simulink model "HDL_source"  (R2019a)
settings: Solver=FixedStepDiscrete  StartTime=0.0  StopTime=0.1  RelTol=1e-3
PreLoadFcn:
  | load('visionhdlLaneDetectionInit.mat');
  | 
  | %Birds-Eye View Parameters:
  | T_unreal = [-0.346719845290643,-3.45626583672944e-16,-2.42608110520569e-19;-1.76272742794994,-2.62399506819665,-0.00185184300876343;1283.14845282490,1569.57420684550,1];
  | shiftleft = single([-5,-5,-5,-5,-5,-5,-5,-5,-5,-5,   -5,-4,-2,-2,-2,-2,0,0,0,1,    1,2,3,4,5,6,7,10,11,13,     15,17,20,22,26,30,33,38,42,46]);
  | shiftright = single([-20,-20,-20,-20,-20,-20,-20,-20,-20,-20,    -20,-20,-20,-21,-22,-23,-24,-24,-24,-25,    -26,-27,-28,-29,-30,-32,-33,-35,-37,-39,    -41,-45,-46,-50,-53,-57,-61,-67,-72,-78]);
StartFcn:
  | warning('off','Coder:MATLAB:polyfit_RepeatedPointsOrRescale');
  | warning('off','Coder:MATLAB:rankDeficientMatrix');
StopFcn:
  | warning('on','Coder:MATLAB:polyfit_RepeatedPointsOrRescale');
  | warning('on','Coder:MATLAB:rankDeficientMatrix');
undefined symbols (not defined in the file): gray, h1, imresize, Rec, SDTV
libraries: simulink x31, hdlsllib x19, visionhdlutilities x6, visionhdlstatistics x4, visiongeotforms x3, visionhdlio x2, visiontextngfix x2, visionhdlconversions x1, visionhdlgeotforms x1, visionhdlfilter x1, dspvision x1, visionsinks x1
(part 2 of 3)

== system HDL_source/FPGALaneDetection/Lane Detection Algorithm/ComputeEgoLanes1/FirstPassEgoLane/rightminop6 ==
  val1 : Inport
  val2 : Inport  Port=2
  ind1 : Inport  Port=3
  ind2 : Inport  Port=4
  Delay{,1..5} (6 alike) : Delay  DelayLength=1
  Multiport Switch : MultiPortSwitch  DataPortOrder=Zero-based contiguous  Inputs=2  zeroidx=on
  Multiport Switch1 : MultiPortSwitch  DataPortOrder=Zero-based contiguous  Inputs=2  zeroidx=on
  Relational Operator : RelationalOperator  Operator=<=  OutDataTypeStr=boolean  RndMeth=Simplest
  valmin : Outport
  indmin : Outport  Port=2
  wires:
  val1/1 -> Delay2/1
  Multiport Switch1/1 -> Delay1/1
  val2/1 -> Delay3/1
  ind1/1 -> Delay4/1
  Multiport Switch/1 -> Delay/1
  Relational Operator/1 -> Multiport Switch/1, Multiport Switch1/1
  ind2/1 -> Delay5/1
  Delay/1 -> valmin/1
  Delay1/1 -> indmin/1
  Delay2/1 -> Relational Operator/1, Multiport Switch/3
  Delay3/1 -> Relational Operator/2, Multiport Switch/2
  Delay4/1 -> Multiport Switch1/3
  Delay5/1 -> Multiport Switch1/2

== system HDL_source/FPGALaneDetection/Lane Detection Algorithm/ComputeEgoLanes1/FirstPassEgoLane/rightminop7 ==
  val1 : Inport
  val2 : Inport  Port=2
  ind1 : Inport  Port=3
  ind2 : Inport  Port=4
  Delay{,1..5} (6 alike) : Delay  DelayLength=1
  Multiport Switch : MultiPortSwitch  DataPortOrder=Zero-based contiguous  Inputs=2  zeroidx=on
  Multiport Switch1 : MultiPortSwitch  DataPortOrder=Zero-based contiguous  Inputs=2  zeroidx=on
  Relational Operator : RelationalOperator  Operator=<=  OutDataTypeStr=boolean  RndMeth=Simplest
  valmin : Outport
  indmin : Outport  Port=2
  wires:
  Delay5/1 -> Multiport Switch1/2
  Delay4/1 -> Multiport Switch1/3
  Delay3/1 -> Multiport Switch/2, Relational Operator/2
  Delay2/1 -> Multiport Switch/3, Relational Operator/1
  Delay1/1 -> indmin/1
  Delay/1 -> valmin/1
  ind2/1 -> Delay5/1
  Relational Operator/1 -> Multiport Switch1/1, Multiport Switch/1
  Multiport Switch/1 -> Delay/1
  ind1/1 -> Delay4/1
  val2/1 -> Delay3/1
  Multiport Switch1/1 -> Delay1/1
  val1/1 -> Delay2/1

== system HDL_source/FPGALaneDetection/Lane Detection Algorithm/ComputeEgoLanes1/FirstPassEgoLane/rightminop8 ==
  val1 : Inport
  val2 : Inport  Port=2
  ind1 : Inport  Port=3
  ind2 : Inport  Port=4
  Delay{,1..5} (6 alike) : Delay  DelayLength=1
  Multiport Switch : MultiPortSwitch  DataPortOrder=Zero-based contiguous  Inputs=2  zeroidx=on
  Multiport Switch1 : MultiPortSwitch  DataPortOrder=Zero-based contiguous  Inputs=2  zeroidx=on
  Relational Operator : RelationalOperator  Operator=<=  OutDataTypeStr=boolean  RndMeth=Simplest
  valmin : Outport
  indmin : Outport  Port=2
  wires:
  val1/1 -> Delay2/1
  Multiport Switch1/1 -> Delay1/1
  val2/1 -> Delay3/1
  ind1/1 -> Delay4/1
  Multiport Switch/1 -> Delay/1
  Relational Operator/1 -> Multiport Switch/1, Multiport Switch1/1
  ind2/1 -> Delay5/1
  Delay/1 -> valmin/1
  Delay1/1 -> indmin/1
  Delay2/1 -> Relational Operator/1, Multiport Switch/3
  Delay3/1 -> Relational Operator/2, Multiport Switch/2
  Delay4/1 -> Multiport Switch1/3
  Delay5/1 -> Multiport Switch1/2

== system HDL_source/FPGALaneDetection/Lane Detection Algorithm/ComputeEgoLanes1/FirstPassEgoLane/rightminop9 ==
  val1 : Inport
  val2 : Inport  Port=2
  ind1 : Inport  Port=3
  ind2 : Inport  Port=4
  Delay{,1..5} (6 alike) : Delay  DelayLength=1
  Multiport Switch : MultiPortSwitch  DataPortOrder=Zero-based contiguous  Inputs=2  zeroidx=on
  Multiport Switch1 : MultiPortSwitch  DataPortOrder=Zero-based contiguous  Inputs=2  zeroidx=on
  Relational Operator : RelationalOperator  Operator=<=  OutDataTypeStr=boolean  RndMeth=Simplest
  valmin : Outport
  indmin : Outport  Port=2
  wires:
  Delay5/1 -> Multiport Switch1/2
  Delay4/1 -> Multiport Switch1/3
  Delay3/1 -> Multiport Switch/2, Relational Operator/2
  Delay2/1 -> Multiport Switch/3, Relational Operator/1
  Delay1/1 -> indmin/1
  Delay/1 -> valmin/1
  ind2/1 -> Delay5/1
  Relational Operator/1 -> Multiport Switch1/1, Multiport Switch/1
  Multiport Switch/1 -> Delay/1
  ind1/1 -> Delay4/1
  val2/1 -> Delay3/1
  Multiport Switch1/1 -> Delay1/1
  val1/1 -> Delay2/1

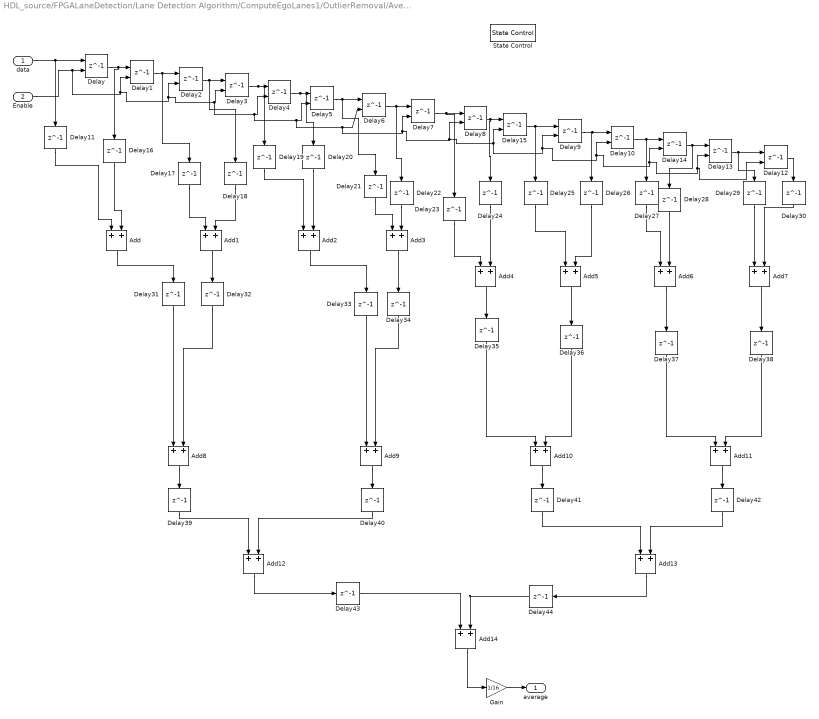
== system HDL_source/FPGALaneDetection/Lane Detection Algorithm/ComputeEgoLanes1/OutlierRemoval/AverageLeftWidth ==
  data : Inport
  Enable : Inport  Port=2
  Add{,1..14} (15 alike) : Sum  OutDataTypeStr=fixdt(1,16,0)
  Delay{,1..10,12..15} (15 alike) : Delay  DelayLength=1  ShowEnablePort=on
      settings: InputPortMap=u0,e6
  Delay{11,16..44} (30 alike) : Delay  DelayLength=1
  Gain : Gain  Gain=1/16
  State Control : StateControl  StateControl=Synchronous
  average : Outport
  wires:
  Delay44/1 -> Add14/2
  Delay43/1 -> Add14/1
  Delay42/1 -> Add13/2
  Delay41/1 -> Add13/1
  Delay40/1 -> Add12/2
  Delay39/1 -> Add12/1
  Delay38/1 -> Add11/2
  Delay37/1 -> Add11/1
  Delay36/1 -> Add10/2
  Delay35/1 -> Add10/1
  Delay34/1 -> Add9/2
  Delay33/1 -> Add9/1
  Delay32/1 -> Add8/2
  Delay31/1 -> Add8/1
  Delay30/1 -> Add7/2
  Delay29/1 -> Add7/1
  Delay28/1 -> Add6/2
  Delay10/1 -> Delay14/1, Delay27/1
  Delay27/1 -> Add6/1
  Delay26/1 -> Add5/2
  Delay25/1 -> Add5/1
  Delay24/1 -> Add4/2
  Delay23/1 -> Add4/1
  Delay22/1 -> Add3/2
  Delay21/1 -> Add3/1
  Delay20/1 -> Add2/2
  Delay19/1 -> Add2/1
  Delay18/1 -> Add1/2
  Delay17/1 -> Add1/1
  Delay16/1 -> Add/2
  Delay11/1 -> Add/1
  Add13/1 -> Delay44/1
  Add12/1 -> Delay43/1
  Add11/1 -> Delay42/1
  Add10/1 -> Delay41/1
  Add9/1 -> Delay40/1
  Add8/1 -> Delay39/1
  Add7/1 -> Delay38/1
  Add6/1 -> Delay37/1
  Add5/1 -> Delay36/1
  Add4/1 -> Delay35/1
  Add3/1 -> Delay34/1
  Add2/1 -> Delay33/1
  Add1/1 -> Delay32/1
  Add/1 -> Delay31/1
  Add14/1 -> Gain/1
  Gain/1 -> average/1
  Delay13/1 -> Delay12/1, Delay29/1
  Delay/1 -> Delay1/1, Delay16/1
  Delay12/1 -> Delay30/1
  Delay14/1 -> Delay13/1, Delay28/1
  Delay9/1 -> Delay10/1, Delay26/1
  Delay15/1 -> Delay9/1, Delay25/1
  Delay8/1 -> Delay15/1, Delay24/1
  Delay7/1 -> Delay8/1, Delay23/1
  Delay6/1 -> Delay7/1, Delay22/1
  Delay5/1 -> Delay6/1, Delay21/1
  Delay4/1 -> Delay20/1, Delay5/1
  Delay3/1 -> Delay4/1, Delay19/1
  Delay2/1 -> Delay3/1, Delay18/1
  Delay1/1 -> Delay2/1, Delay17/1
  Enable/1 -> Delay/2, Delay1/2, Delay2/2, Delay3/2, Delay4/2, Delay5/2, Delay6/2, Delay7/2, Delay8/2, Delay9/2, Delay10/2, Delay14/2, Delay13/2, Delay12/2, Delay15/2
  data/1 -> Delay/1, Delay11/1

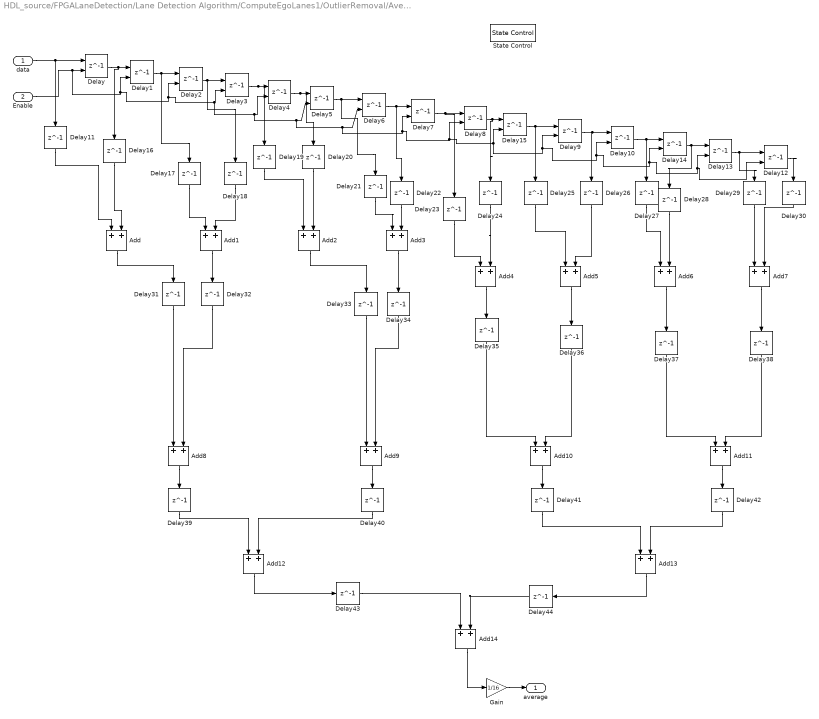
== system HDL_source/FPGALaneDetection/Lane Detection Algorithm/ComputeEgoLanes1/OutlierRemoval/AverageRightWidth ==
  data : Inport
  Enable : Inport  Port=2
  Add{,1..14} (15 alike) : Sum  OutDataTypeStr=fixdt(1,16,0)
  Delay{,1..10,12..15} (15 alike) : Delay  DelayLength=1  ShowEnablePort=on
      settings: InputPortMap=u0,e6
  Delay{11,16..44} (30 alike) : Delay  DelayLength=1
  Gain : Gain  Gain=1/16
  State Control : StateControl  StateControl=Synchronous
  average : Outport
  wires:
  data/1 -> Delay11/1, Delay/1
  Enable/1 -> Delay15/2, Delay12/2, Delay13/2, Delay14/2, Delay10/2, Delay9/2, Delay8/2, Delay7/2, Delay6/2, Delay5/2, Delay4/2, Delay3/2, Delay2/2, Delay1/2, Delay/2
  Delay1/1 -> Delay17/1, Delay2/1
  Delay2/1 -> Delay18/1, Delay3/1
  Delay3/1 -> Delay19/1, Delay4/1
  Delay4/1 -> Delay20/1, Delay5/1
  Delay5/1 -> Delay21/1, Delay6/1
  Delay6/1 -> Delay22/1, Delay7/1
  Delay7/1 -> Delay23/1, Delay8/1
  Delay8/1 -> Delay24/1, Delay15/1
  Delay15/1 -> Delay25/1, Delay9/1
  Delay9/1 -> Delay26/1, Delay10/1
  Delay14/1 -> Delay28/1, Delay13/1
  Delay12/1 -> Delay30/1
  Delay/1 -> Delay16/1, Delay1/1
  Delay13/1 -> Delay29/1, Delay12/1
  Gain/1 -> average/1
  Add14/1 -> Gain/1
  Add/1 -> Delay31/1
  Add1/1 -> Delay32/1
  Add2/1 -> Delay33/1
  Add3/1 -> Delay34/1
  Add4/1 -> Delay35/1
  Add5/1 -> Delay36/1
  Add6/1 -> Delay37/1
  Add7/1 -> Delay38/1
  Add8/1 -> Delay39/1
  Add9/1 -> Delay40/1
  Add10/1 -> Delay41/1
  Add11/1 -> Delay42/1
  Add12/1 -> Delay43/1
  Add13/1 -> Delay44/1
  Delay11/1 -> Add/1
  Delay16/1 -> Add/2
  Delay17/1 -> Add1/1
  Delay18/1 -> Add1/2
  Delay19/1 -> Add2/1
  Delay20/1 -> Add2/2
  Delay21/1 -> Add3/1
  Delay22/1 -> Add3/2
  Delay23/1 -> Add4/1
  Delay24/1 -> Add4/2
  Delay25/1 -> Add5/1
  Delay26/1 -> Add5/2
  Delay27/1 -> Add6/1
  Delay10/1 -> Delay27/1, Delay14/1
  Delay28/1 -> Add6/2
  Delay29/1 -> Add7/1
  Delay30/1 -> Add7/2
  Delay31/1 -> Add8/1
  Delay32/1 -> Add8/2
  Delay33/1 -> Add9/1
  Delay34/1 -> Add9/2
  Delay35/1 -> Add10/1
  Delay36/1 -> Add10/2
  Delay37/1 -> Add11/1
  Delay38/1 -> Add11/2
  Delay39/1 -> Add12/1
  Delay40/1 -> Add12/2
  Delay41/1 -> Add13/1
  Delay42/1 -> Add13/2
  Delay43/1 -> Add14/1
  Delay44/1 -> Add14/2

== system HDL_source/FPGALaneDetection/Lane Detection Algorithm/ComputeEgoLanes1/OutlierRemoval/RemoveOutlier ==
  laneVal : Inport
  offsetVal : Inport  Port=2
  width : Inport  Port=3
  Constant2 : Constant  Value=0  OutDataTypeStr=uint16  SampleTime=-1
  Delay{13..15,17} (4 alike) : Delay  DelayLength=1
  Multiport Switch : MultiPortSwitch  DataPortOrder=Zero-based contiguous  Inputs=2  zeroidx=on
  Relational Operator : RelationalOperator  Operator=<=  OutDataTypeStr=boolean  RndMeth=Simplest
  Inlier : Outport
  wires:
  Delay14/1 -> Multiport Switch/2
  Multiport Switch/1 -> Delay17/1
  Delay15/1 -> Multiport Switch/3
  Relational Operator/1 -> Delay13/1
  offsetVal/1 -> Relational Operator/1
  laneVal/1 -> Delay15/1
  Constant2/1 -> Delay14/1
  Delay13/1 -> Multiport Switch/1
  width/1 -> Relational Operator/2
  Delay17/1 -> Inlier/1

== system HDL_source/FPGALaneDetection/Lane Detection Algorithm/ComputeEgoLanes1/OutlierRemoval/RemoveOutlier1 ==
  laneVal : Inport
  offsetVal : Inport  Port=2
  width : Inport  Port=3
  Constant2 : Constant  Value=0  OutDataTypeStr=uint16  SampleTime=-1
  Delay{13..15,17} (4 alike) : Delay  DelayLength=1
  Multiport Switch : MultiPortSwitch  DataPortOrder=Zero-based contiguous  Inputs=2  zeroidx=on
  Relational Operator : RelationalOperator  Operator=<=  OutDataTypeStr=boolean  RndMeth=Simplest
  Inlier : Outport
  wires:
  Delay17/1 -> Inlier/1
  width/1 -> Relational Operator/2
  Delay13/1 -> Multiport Switch/1
  Constant2/1 -> Delay14/1
  laneVal/1 -> Delay15/1
  offsetVal/1 -> Relational Operator/1
  Relational Operator/1 -> Delay13/1
  Delay15/1 -> Multiport Switch/3
  Multiport Switch/1 -> Delay17/1
  Delay14/1 -> Multiport Switch/2

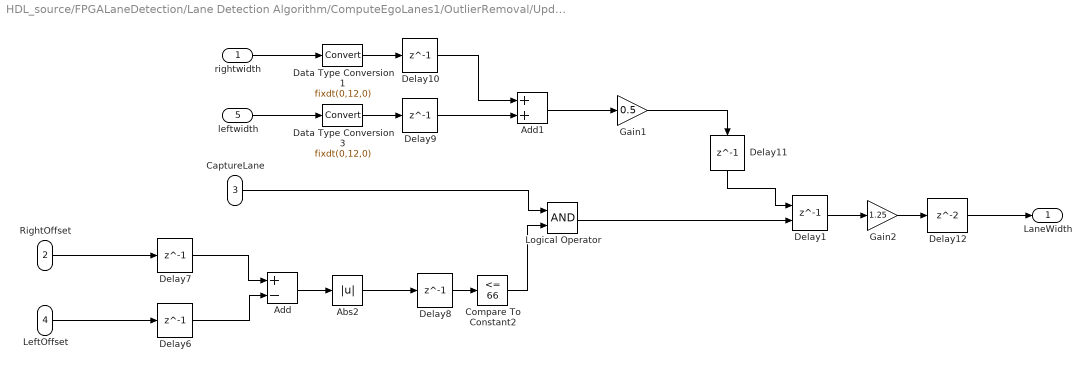
== system HDL_source/FPGALaneDetection/Lane Detection Algorithm/ComputeEgoLanes1/OutlierRemoval/UpdateLaneWidth ==
  rightwidth : Inport
  RightOffset : Inport  Port=2
  CaptureLane : Inport  Port=3
  LeftOffset : Inport  Port=4
  leftwidth : Inport  Port=5
  Abs2 : Abs  OutDataTypeStr=fixdt(0,14,0)
  Add : Sum  Inputs=+-  SaturateOnIntegerOverflow=on
  Add1 : Sum
  Compare To Constant2 : simulink/Logic and Bit Operations/Compare To Constant  relop=<=  const=66  OutDataTypeStr=boolean
  Data Type Conversion1 : DataTypeConversion  OutDataTypeStr=fixdt(0,12,0)  RndMeth=Round  SaturateOnIntegerOverflow=on
  Data Type Conversion3 : DataTypeConversion  OutDataTypeStr=fixdt(0,12,0)  RndMeth=Round  SaturateOnIntegerOverflow=on
  Delay1 : Delay  DelayLength=1  ShowEnablePort=on
      settings: InputPortMap=u0,e6
  Delay{6..11} (6 alike) : Delay  DelayLength=1
  Delay12 : Delay
  Gain1 : Gain  Gain=0.5  OutDataTypeStr=fixdt(0,16,0)  RndMeth=Round  SaturateOnIntegerOverflow=on
  Gain2 : Gain  Gain=1.25  OutDataTypeStr=fixdt(1,18,0)
  Logical Operator : Logic  AllPortsSameDT=off  OutDataTypeStr=boolean
  LaneWidth : Outport
  wires:
  Compare To Constant2/1 -> Logical Operator/2
  Gain1/1 -> Delay11/1
  Abs2/1 -> Delay8/1
  Delay8/1 -> Compare To Constant2/1
  LeftOffset/1 -> Delay6/1
  Delay10/1 -> Add1/1
  Delay11/1 -> Delay1/1
  rightwidth/1 -> Data Type Conversion1/1
  leftwidth/1 -> Data Type Conversion3/1
  Delay7/1 -> Add/1
  CaptureLane/1 -> Logical Operator/1
  Add/1 -> Abs2/1
  Delay12/1 -> LaneWidth/1
  Delay9/1 -> Add1/2
  Delay1/1 -> Gain2/1
  Add1/1 -> Gain1/1
  Logical Operator/1 -> Delay1/2
  Delay6/1 -> Add/2
  Gain2/1 -> Delay12/1
  RightOffset/1 -> Delay7/1
  Data Type Conversion1/1 -> Delay10/1
  Data Type Conversion3/1 -> Delay9/1

== system HDL_source/FPGALaneDetection/Lane Detection Algorithm/LaneDetection1/LaneCandidateGeneration/HistogramColumnCount ==
  pixelIn : Inport
  controlIn : Inport  Port=2
  ColumnCountNeg : Subsystem
  ColumnCountPos : Subsystem
  Compare To Constant : simulink/Logic and Bit Operations/Compare To Constant  relop=>  const=0.8  OutDataTypeStr=boolean
  Compare To Constant1 : simulink/Logic and Bit Operations/Compare To Constant  relop=<  const=-0.8  OutDataTypeStr=boolean
  PositiveHistogramCount : Outport
  HistogramValid : Outport  Port=2
  HistogramAddress : Outport  Port=3
  NegativeHistogramCount : Outport  Port=4
  wires:
  controlIn/1 -> ColumnCountPos/2(controlIn), ColumnCountNeg/2(controlIn)
  Compare To Constant/1 -> ColumnCountPos/1(pixelIn)
  pixelIn/1 -> Compare To Constant/1, Compare To Constant1/1
  ColumnCountPos/3(HistogramAddress) -> HistogramAddress/1
  ColumnCountNeg/1(NegativeHistogramCount) -> NegativeHistogramCount/1
  ColumnCountPos/1(PositiveHistogramCount) -> PositiveHistogramCount/1
  Compare To Constant1/1 -> ColumnCountNeg/1(pixelIn)
  ColumnCountPos/2(HistogramValid) -> HistogramValid/1

== system HDL_source/FPGALaneDetection/Lane Detection Algorithm/LaneDetection1/LaneCandidateGeneration/OverlapandMultiply ==
  note: offset columns
  note: pipelining
  posHistCount : Inport
  negHistCount : Inport  Port=2
  Delay1 : Delay
  Delay2 : Delay
  Delay3 : Delay
  Delay8 : Delay  DelayLength=18
  Product : Product  RndMeth=Round  SaturateOnIntegerOverflow=on
  matchedHist : Outport
  wires:
  Delay3/1 -> matchedHist/1
  posHistCount/1 -> Delay8/1
  Delay1/1 -> Product/1
  Delay8/1 -> Delay1/1
  negHistCount/1 -> Delay2/1
  Delay2/1 -> Product/2
  Product/1 -> Delay3/1

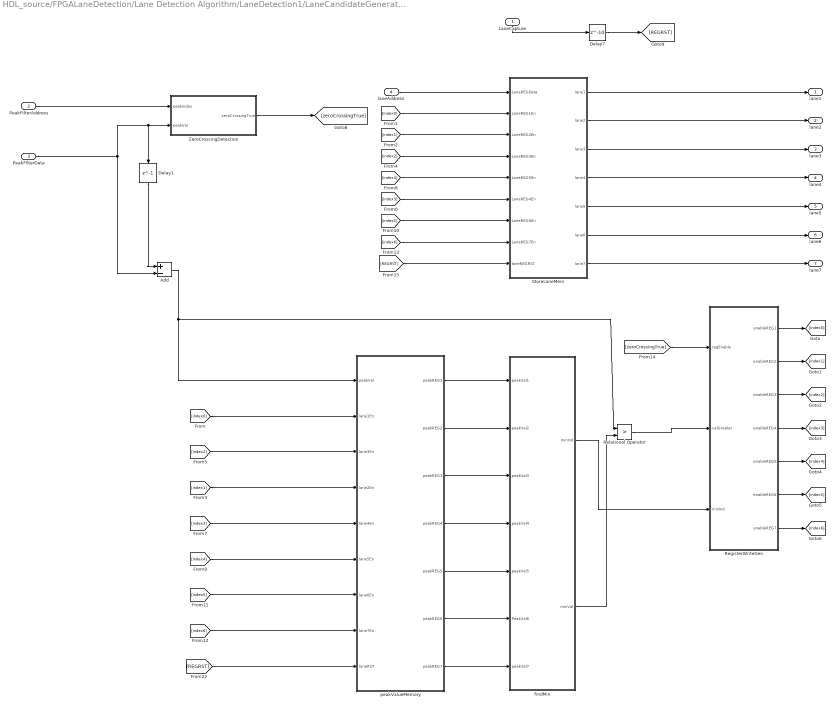
== system HDL_source/FPGALaneDetection/Lane Detection Algorithm/LaneDetection1/LaneCandidateGeneration/StoreDominantLanes ==
  LaneCapture : Inport
  PeakFIlterAddress : Inport  Port=2
  PeakFIlterData : Inport  Port=3
  laneAddress : Inport  Port=4
  Add : Sum  Inputs=+-  SaturateOnIntegerOverflow=on
  Delay1 : Delay  DelayLength=1
  Delay7 : Delay  DelayLength=10
  RegisterWriteGen : Subsystem
  Relational Operator : RelationalOperator  Operator=>  OutDataTypeStr=boolean  RndMeth=Nearest
  StoreLaneMem : Subsystem
  ZeroCrossingDetection : Subsystem
  findMin : Subsystem
  peakValueMemory : Subsystem
  lane1 : Outport
  lane2 : Outport  Port=2
  lane3 : Outport  Port=3
  lane4 : Outport  Port=4
  lane5 : Outport  Port=5
  lane6 : Outport  Port=6
  lane7 : Outport  Port=7
  wires:
  LaneCapture/1 -> Delay7/1
  PeakFIlterAddress/1 -> ZeroCrossingDetection/1(peakIndex)
  laneAddress/1 -> StoreLaneMem/1(LaneREGData)
  StoreLaneMem/7(lane7) -> lane7/1
  StoreLaneMem/6(lane6) -> lane6/1
  StoreLaneMem/5(lane5) -> lane5/1
  StoreLaneMem/4(lane4) -> lane4/1
  StoreLaneMem/3(lane3) -> lane3/1
  StoreLaneMem/2(lane2) -> lane2/1
  StoreLaneMem/1(lane1) -> lane1/1
  [index6] -> StoreLaneMem/8(LaneREG7En)
  [index5] -> StoreLaneMem/7(LaneREG6En)
  [index3] -> StoreLaneMem/6(LaneREG4En)
  [index4] -> StoreLaneMem/5(LaneREG5En)
  [index2] -> StoreLaneMem/4(LaneREG3En)
  [index1] -> StoreLaneMem/3(LaneREG2En)
  [REGRST] -> StoreLaneMem/9(laneREGRST)
  [index0] -> StoreLaneMem/2(LaneREG1En)
  Delay1/1 -> Add/1
  ZeroCrossingDetection/1(zeroCrossingTrue) -> [zeroCrossingTrue]
  peakValueMemory/7(peakREG7) -> findMin/7(peakVal7)
  peakValueMemory/6(peakREG6) -> findMin/6(PeakVal6)
  peakValueMemory/5(peakREG5) -> findMin/5(peakVal5)
  peakValueMemory/4(peakREG4) -> findMin/4(peakVal4)
  peakValueMemory/3(peakREG3) -> findMin/3(peakVal3)
  peakValueMemory/2(peakREG2) -> findMin/2(peakVal2)
  peakValueMemory/1(peakREG1) -> findMin/1(peakVal1)
  [index6] -> peakValueMemory/8(lane7En)
  [index5] -> peakValueMemory/7(lane6En)
  [index4] -> peakValueMemory/6(lane5En)
  [index3] -> peakValueMemory/5(lane4En)
  [index1] -> peakValueMemory/4(lane2En)
  [REGRST] -> peakValueMemory/9(laneRST)
  [index2] -> peakValueMemory/3(lane3En)
  [index0] -> peakValueMemory/2(lane1En)
  RegisterWriteGen/7(enableREG7) -> [index6]
  RegisterWriteGen/6(enableREG6) -> [index5]
  RegisterWriteGen/5(enableREG5) -> [index4]
  RegisterWriteGen/4(enableREG4) -> [index3]
  RegisterWriteGen/3(enableREG3) -> [index2]
  RegisterWriteGen/2(enableREG2) -> [index1]
  RegisterWriteGen/1(enableREG1) -> [index0]
  findMin/1(minInd) -> RegisterWriteGen/3(minInd)
  Relational Operator/1 -> RegisterWriteGen/2(valGreater)
  [zeroCrossingTrue] -> RegisterWriteGen/1(regEnable)
  Add/1 -> Relational Operator/1, peakValueMemory/1(peakVal)
  Delay7/1 -> [REGRST]
  findMin/2(minVal) -> Relational Operator/2
  PeakFIlterData/1 -> Add/2, ZeroCrossingDetection/2(peakVal), Delay1/1

== system HDL_source/FPGALaneDetection/Lane Detection Algorithm/LaneDetection1/LaneCandidateGeneration/ZeroCrossingFilter ==
  In1 : Inport
  In2 : Inport  Port=2
  Data Type Conversion1 : DataTypeConversion  OutDataTypeStr=fixdt(1,14,0)
  Discrete FIR Filter : DiscreteFir  Coefficients=[1:4,-4:-1]  ShowEnablePort=on  RndMeth=Round  SaturateOnIntegerOverflow=on
      settings: InputPortMap=u0,e7
  Out1 : Outport
  wires:
  Data Type Conversion1/1 -> Discrete FIR Filter/1
  In1/1 -> Data Type Conversion1/1
  In2/1 -> Discrete FIR Filter/2
  Discrete FIR Filter/1 -> Out1/1

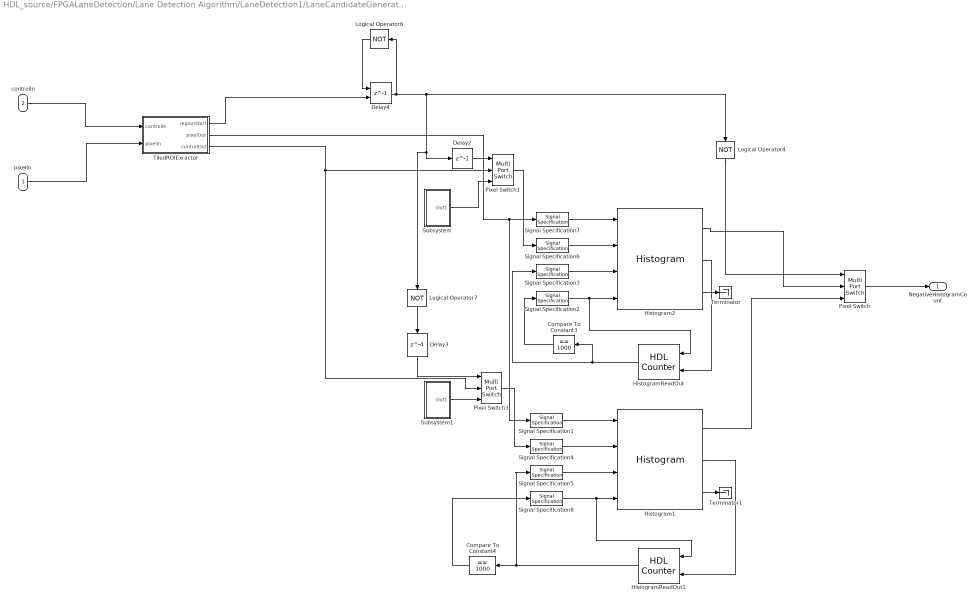
== system HDL_source/FPGALaneDetection/Lane Detection Algorithm/LaneDetection1/LaneCandidateGeneration/HistogramColumnCount/ColumnCountNeg ==
  pixelIn : Inport
  controlIn : Inport  Port=2
  Compare To Constant3 : simulink/Logic and Bit Operations/Compare To Constant  relop===  const=1000  OutDataTypeStr=boolean
  Compare To Constant4 : simulink/Logic and Bit Operations/Compare To Constant  relop===  const=1000  OutDataTypeStr=boolean
  Delay2 : Delay  DelayLength=1
  Delay3 : Delay  DelayLength=4
  Delay4 : Delay  DelayLength=1  ShowEnablePort=on
      settings: InputPortMap=u0,e6
  Histogram1 : visionhdlstatistics/Histogram  NumBins=1024  OutputDataType=Unsigned fixed point  OutputWL=10  SimulateUsing=Code generation
      settings: SourceProductName=Vision HDL Toolbox  SourceProductBaseCode=VT
  Histogram2 : visionhdlstatistics/Histogram  NumBins=1024  OutputDataType=Unsigned fixed point  OutputWL=10  SimulateUsing=Code generation
      settings: SourceProductName=Vision HDL Toolbox  SourceProductBaseCode=VT
  HistogramReadOut : hdlsllib/Sources/HDL Counter  CountType=Free running  CountInit=0  CountStep=1  CountMax=17  CountFromType=Initial value  CountFrom=0  CountResetPort=on  CountLoadPort=off  CountEnbPort=on  CountDirPort=off  CountDataType=Unsigned  CountWordLen=10  CountFracLen=0  CountSampTime=1
      settings: SourceProductName=Simulink
  HistogramReadOut1 : hdlsllib/Sources/HDL Counter  CountType=Free running  CountInit=0  CountStep=1  CountMax=17  CountFromType=Initial value  CountFrom=0  CountResetPort=on  CountLoadPort=off  CountEnbPort=on  CountDirPort=off  CountDataType=Unsigned  CountWordLen=10  CountFracLen=0  CountSampTime=1
      settings: SourceProductName=Simulink
  Logical Operator4 : Logic  Operator=NOT  AllPortsSameDT=off  OutDataTypeStr=boolean
  Logical Operator6 : Logic  Operator=NOT  AllPortsSameDT=off  OutDataTypeStr=boolean
  Logical Operator7 : Logic  Operator=NOT  AllPortsSameDT=off  OutDataTypeStr=boolean
  Pixel Switch : MultiPortSwitch  DataPortOrder=Zero-based contiguous  Inputs=2  zeroidx=on
  Pixel Switch1 : MultiPortSwitch  DataPortOrder=Zero-based contiguous  Inputs=2  zeroidx=on
  Pixel Switch3 : MultiPortSwitch  DataPortOrder=Zero-based contiguous  Inputs=2  zeroidx=on
  Signal Specification{1..8} (8 alike) : SignalSpecification  Dimensions=1
  Subsystem : Subsystem
  Subsystem1 : Subsystem
  Terminator : Terminator
  Terminator1 : Terminator
  TiledROIExractor : Subsystem
  NegativeHistogramCount : Outport
  wires:
  Histogram2/2 -> HistogramReadOut/2
  Logical Operator6/1 -> Delay4/1
  Pixel Switch3/1 -> Signal Specification4/1
  Histogram2/1 -> Pixel Switch/2
  Pixel Switch/1 -> NegativeHistogramCount/1
  Histogram1/2 -> HistogramReadOut1/2
  Signal Specification5/1 -> Histogram1/3
  Signal Specification8/1 -> HistogramReadOut1/1, Histogram1/4
  Signal Specification2/1 -> Histogram2/4, HistogramReadOut/1
  Signal Specification3/1 -> Histogram2/3
  Signal Specification1/1 -> Histogram1/1
  Signal Specification4/1 -> Histogram1/2
  Signal Specification6/1 -> Histogram2/2
  Signal Specification7/1 -> Histogram2/1
  Logical Operator4/1 -> Pixel Switch/1
  Subsystem/1(Out1) -> Pixel Switch1/3
  Pixel Switch1/1 -> Signal Specification6/1
  Delay2/1 -> Pixel Switch1/1
  Delay4/1 -> Logical Operator4/1, Logical Operator7/1, Delay2/1, Logical Operator6/1
  Subsystem1/1(Out1) -> Pixel Switch3/3
  Logical Operator7/1 -> Delay3/1
  Delay3/1 -> Pixel Switch3/1
  Histogram1/1 -> Pixel Switch/3
  Histogram2/3 -> Terminator/1
  Histogram1/3 -> Terminator1/1
  controlIn/1 -> TiledROIExractor/1(controlIn)
  pixelIn/1 -> TiledROIExractor/2(pixelIn)
  TiledROIExractor/1(regionStart) -> Delay4/2
  TiledROIExractor/3(controlOut) -> Pixel Switch3/2, Pixel Switch1/2
  TiledROIExractor/2(pixelOut) -> Signal Specification1/1, Signal Specification7/1
  Compare To Constant3/1 -> Signal Specification2/1
  HistogramReadOut/1 -> Signal Specification3/1, Compare To Constant3/1
  Compare To Constant4/1 -> Signal Specification8/1
  HistogramReadOut1/1 -> Signal Specification5/1, Compare To Constant4/1

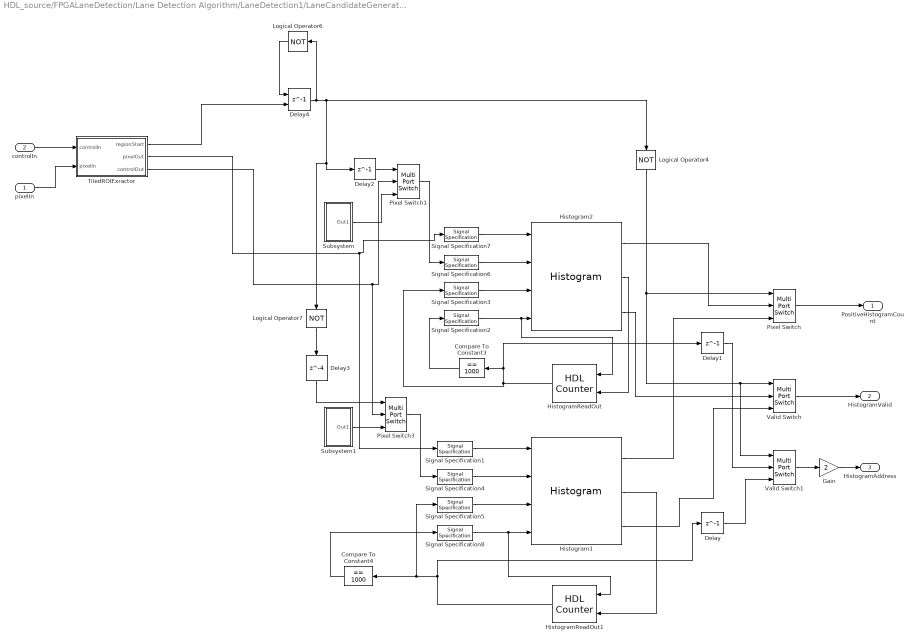
== system HDL_source/FPGALaneDetection/Lane Detection Algorithm/LaneDetection1/LaneCandidateGeneration/HistogramColumnCount/ColumnCountPos ==
  pixelIn : Inport
  controlIn : Inport  Port=2
  Compare To Constant3 : simulink/Logic and Bit Operations/Compare To Constant  relop===  const=1000  OutDataTypeStr=boolean
  Compare To Constant4 : simulink/Logic and Bit Operations/Compare To Constant  relop===  const=1000  OutDataTypeStr=boolean
  Delay : Delay  DelayLength=1
  Delay1 : Delay  DelayLength=1
  Delay2 : Delay  DelayLength=1
  Delay3 : Delay  DelayLength=4
  Delay4 : Delay  DelayLength=1  ShowEnablePort=on
      settings: InputPortMap=u0,e6
  Gain : Gain  Gain=2  OutDataTypeStr=fixdt(0,11,0)
  Histogram1 : visionhdlstatistics/Histogram  NumBins=1024  OutputDataType=Unsigned fixed point  OutputWL=10  SimulateUsing=Code generation
      settings: SourceProductName=Vision HDL Toolbox  SourceProductBaseCode=VT
  Histogram2 : visionhdlstatistics/Histogram  NumBins=1024  OutputDataType=Unsigned fixed point  OutputWL=10  SimulateUsing=Code generation
      settings: SourceProductName=Vision HDL Toolbox  SourceProductBaseCode=VT
  HistogramReadOut : hdlsllib/Sources/HDL Counter  CountType=Free running  CountInit=0  CountStep=1  CountMax=17  CountFromType=Initial value  CountFrom=0  CountResetPort=on  CountLoadPort=off  CountEnbPort=on  CountDirPort=off  CountDataType=Unsigned  CountWordLen=10  CountFracLen=0  CountSampTime=1
      settings: SourceProductName=Simulink
  HistogramReadOut1 : hdlsllib/Sources/HDL Counter  CountType=Free running  CountInit=0  CountStep=1  CountMax=17  CountFromType=Initial value  CountFrom=0  CountResetPort=on  CountLoadPort=off  CountEnbPort=on  CountDirPort=off  CountDataType=Unsigned  CountWordLen=10  CountFracLen=0  CountSampTime=1
      settings: SourceProductName=Simulink
  Logical Operator4 : Logic  Operator=NOT  AllPortsSameDT=off  OutDataTypeStr=boolean
  Logical Operator6 : Logic  Operator=NOT  AllPortsSameDT=off  OutDataTypeStr=boolean
  Logical Operator7 : Logic  Operator=NOT  AllPortsSameDT=off  OutDataTypeStr=boolean
  Pixel Switch : MultiPortSwitch  DataPortOrder=Zero-based contiguous  Inputs=2  zeroidx=on
  Pixel Switch1 : MultiPortSwitch  DataPortOrder=Zero-based contiguous  Inputs=2  zeroidx=on
  Pixel Switch3 : MultiPortSwitch  DataPortOrder=Zero-based contiguous  Inputs=2  zeroidx=on
  Signal Specification{1..8} (8 alike) : SignalSpecification  Dimensions=1
  Subsystem : Subsystem
  Subsystem1 : Subsystem
  TiledROIExractor : Subsystem
  Valid Switch : MultiPortSwitch  DataPortOrder=Zero-based contiguous  Inputs=2  zeroidx=on
  Valid Switch1 : MultiPortSwitch  DataPortOrder=Zero-based contiguous  Inputs=2  zeroidx=on
  PositiveHistogramCount : Outport
  HistogramValid : Outport  Port=2
  HistogramAddress : Outport  Port=3
  wires:
  Histogram1/1 -> Pixel Switch/3
  Delay3/1 -> Pixel Switch3/1
  Logical Operator7/1 -> Delay3/1
  Subsystem1/1(Out1) -> Pixel Switch3/3
  Delay4/1 -> Logical Operator6/1, Delay2/1, Logical Operator7/1, Logical Operator4/1
  Delay2/1 -> Pixel Switch1/1
  Pixel Switch1/1 -> Signal Specification6/1
  Subsystem/1(Out1) -> Pixel Switch1/3
  Logical Operator4/1 -> Valid Switch/1, Valid Switch1/1, Pixel Switch/1
  Delay/1 -> Valid Switch1/3
  Delay1/1 -> Valid Switch1/2
  Valid Switch1/1 -> Gain/1
  Signal Specification7/1 -> Histogram2/1
  Signal Specification6/1 -> Histogram2/2
  Signal Specification4/1 -> Histogram1/2
  Signal Specification1/1 -> Histogram1/1
  Signal Specification3/1 -> Histogram2/3
  Signal Specification2/1 -> Histogram2/4, HistogramReadOut/1
  Signal Specification8/1 -> Histogram1/4, HistogramReadOut1/1
  Signal Specification5/1 -> Histogram1/3
  Histogram1/2 -> HistogramReadOut1/2
  Pixel Switch/1 -> PositiveHistogramCount/1
  Histogram2/1 -> Pixel Switch/2
  Pixel Switch3/1 -> Signal Specification4/1
  Logical Operator6/1 -> Delay4/1
  Histogram2/2 -> HistogramReadOut/2
  Histogram1/3 -> Valid Switch/3
  Valid Switch/1 -> HistogramValid/1
  Histogram2/3 -> Valid Switch/2
  TiledROIExractor/2(pixelOut) -> Signal Specification1/1, Signal Specification7/1
  TiledROIExractor/3(controlOut) -> Pixel Switch1/2, Pixel Switch3/2
  controlIn/1 -> TiledROIExractor/1(controlIn)
  pixelIn/1 -> TiledROIExractor/2(pixelIn)
  TiledROIExractor/1(regionStart) -> Delay4/2
  HistogramReadOut/1 -> Signal Specification3/1, Compare To Constant3/1, Delay1/1
  Compare To Constant3/1 -> Signal Specification2/1
  Compare To Constant4/1 -> Signal Specification8/1
  HistogramReadOut1/1 -> Delay/1, Signal Specification5/1, Compare To Constant4/1
  Gain/1 -> HistogramAddress/1

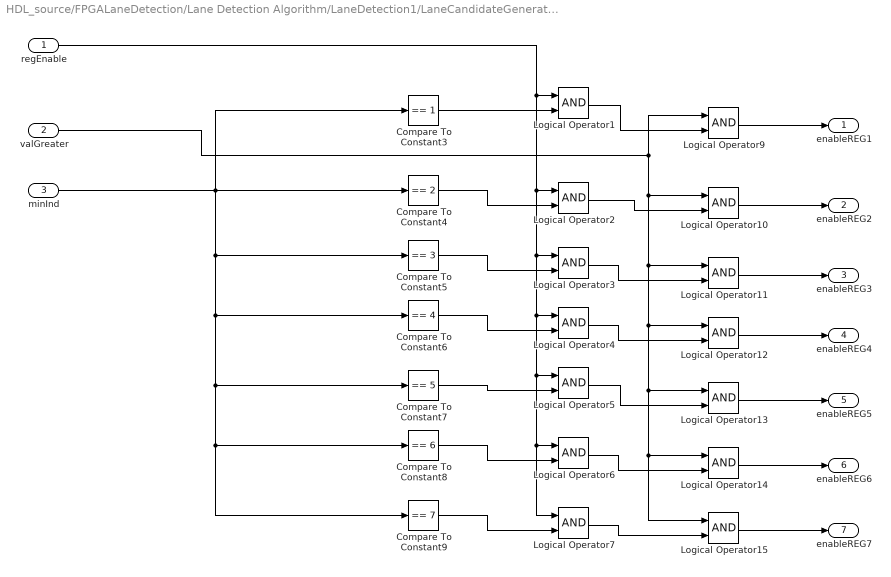
== system HDL_source/FPGALaneDetection/Lane Detection Algorithm/LaneDetection1/LaneCandidateGeneration/StoreDominantLanes/RegisterWriteGen ==
  regEnable : Inport
  valGreater : Inport  Port=2
  minInd : Inport  Port=3
  Compare To Constant3 : simulink/Logic and Bit Operations/Compare To Constant  relop===  const=1  OutDataTypeStr=boolean
  Compare To Constant4 : simulink/Logic and Bit Operations/Compare To Constant  relop===  const=2  OutDataTypeStr=boolean
  Compare To Constant5 : simulink/Logic and Bit Operations/Compare To Constant  relop===  const=3  OutDataTypeStr=boolean
  Compare To Constant6 : simulink/Logic and Bit Operations/Compare To Constant  relop===  const=4  OutDataTypeStr=boolean
  Compare To Constant7 : simulink/Logic and Bit Operations/Compare To Constant  relop===  const=5  OutDataTypeStr=boolean
  Compare To Constant8 : simulink/Logic and Bit Operations/Compare To Constant  relop===  const=6  OutDataTypeStr=boolean
  Compare To Constant9 : simulink/Logic and Bit Operations/Compare To Constant  relop===  const=7  OutDataTypeStr=boolean
  Logical Operator{1..7,9..15} (14 alike) : Logic  AllPortsSameDT=off  OutDataTypeStr=boolean
  enableREG1 : Outport
  enableREG2 : Outport  Port=2
  enableREG3 : Outport  Port=3
  enableREG4 : Outport  Port=4
  enableREG5 : Outport  Port=5
  enableREG6 : Outport  Port=6
  enableREG7 : Outport  Port=7
  wires:
  valGreater/1 -> Logical Operator10/1, Logical Operator11/1, Logical Operator12/1, Logical Operator13/1, Logical Operator14/1, Logical Operator15/1, Logical Operator9/1
  Logical Operator5/1 -> Logical Operator13/2
  Compare To Constant4/1 -> Logical Operator2/2
  Compare To Constant3/1 -> Logical Operator1/2
  Compare To Constant6/1 -> Logical Operator4/2
  Compare To Constant5/1 -> Logical Operator3/2
  Logical Operator2/1 -> Logical Operator10/2
  Logical Operator9/1 -> enableREG1/1
  minInd/1 -> Compare To Constant4/1, Compare To Constant5/1, Compare To Constant6/1, Compare To Constant7/1, Compare To Constant8/1, Compare To Constant9/1, Compare To Constant3/1
  Logical Operator3/1 -> Logical Operator11/2
  Logical Operator1/1 -> Logical Operator9/2
  Logical Operator4/1 -> Logical Operator12/2
  Logical Operator11/1 -> enableREG3/1
  Compare To Constant7/1 -> Logical Operator5/2
  Logical Operator6/1 -> Logical Operator14/2
  Logical Operator14/1 -> enableREG6/1
  Logical Operator10/1 -> enableREG2/1
  Logical Operator13/1 -> enableREG5/1
  regEnable/1 -> Logical Operator1/1, Logical Operator2/1, Logical Operator3/1, Logical Operator4/1, Logical Operator5/1, Logical Operator6/1, Logical Operator7/1
  Logical Operator12/1 -> enableREG4/1
  Logical Operator7/1 -> Logical Operator15/2
  Compare To Constant9/1 -> Logical Operator7/2
  Compare To Constant8/1 -> Logical Operator6/2
  Logical Operator15/1 -> enableREG7/1

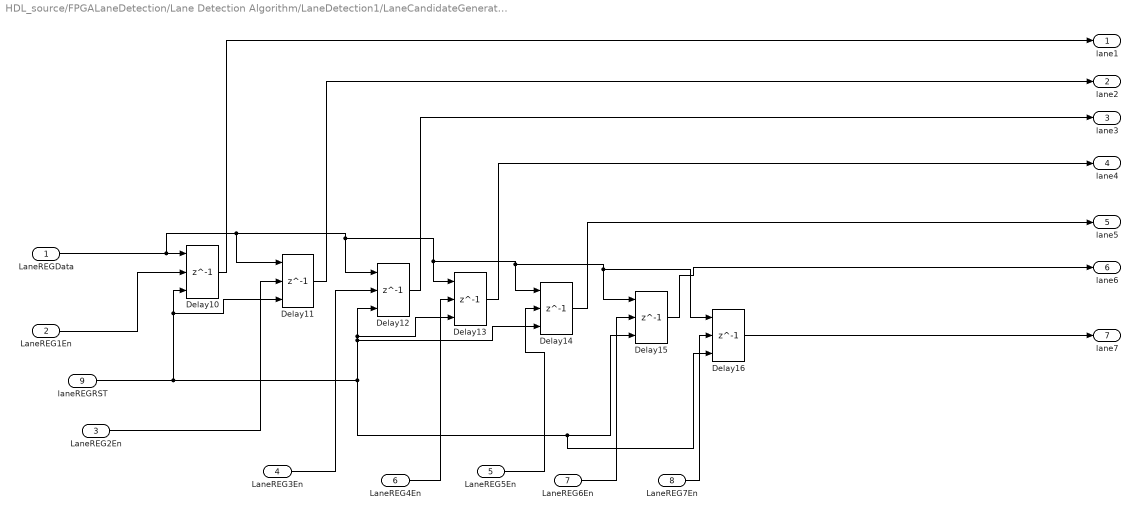
== system HDL_source/FPGALaneDetection/Lane Detection Algorithm/LaneDetection1/LaneCandidateGeneration/StoreDominantLanes/StoreLaneMem ==
  LaneREGData : Inport
  LaneREG1En : Inport  Port=2
  LaneREG2En : Inport  Port=3
  LaneREG3En : Inport  Port=4
  LaneREG5En : Inport  Port=5
  LaneREG4En : Inport  Port=6
  LaneREG6En : Inport  Port=7
  LaneREG7En : Inport  Port=8
  laneREGRST : Inport  Port=9
  Delay{10..16} (7 alike) : Delay  DelayLength=1  ExternalReset=Level hold  ShowEnablePort=on
      settings: InputPortMap=u0,e6,r5
  lane1 : Outport
  lane2 : Outport  Port=2
  lane3 : Outport  Port=3
  lane4 : Outport  Port=4
  lane5 : Outport  Port=5
  lane6 : Outport  Port=6
  lane7 : Outport  Port=7
  wires:
  laneREGRST/1 -> Delay10/3, Delay11/3, Delay15/3, Delay16/3, Delay12/3, Delay13/3, Delay14/3
  LaneREG2En/1 -> Delay11/2
  Delay10/1 -> lane1/1
  LaneREG5En/1 -> Delay14/2
  LaneREG1En/1 -> Delay10/2
  LaneREG7En/1 -> Delay16/2
  Delay16/1 -> lane7/1
  Delay15/1 -> lane6/1
  LaneREG3En/1 -> Delay12/2
  LaneREG6En/1 -> Delay15/2
  Delay12/1 -> lane3/1
  Delay13/1 -> lane4/1
  LaneREG4En/1 -> Delay13/2
  Delay14/1 -> lane5/1
  LaneREGData/1 -> Delay15/1, Delay16/1, Delay14/1, Delay13/1, Delay12/1, Delay11/1, Delay10/1
  Delay11/1 -> lane2/1

== system HDL_source/FPGALaneDetection/Lane Detection Algorithm/LaneDetection1/LaneCandidateGeneration/StoreDominantLanes/ZeroCrossingDetection ==
  peakIndex : Inport
  peakVal : Inport  Port=2
  Compare To Constant11 : simulink/Logic and Bit Operations/Compare To Constant  relop=<  const=1920  OutDataTypeStr=boolean
  Compare To Constant12 : simulink/Logic and Bit Operations/Compare To Constant  relop=>  const=5  OutDataTypeStr=boolean
  Compare To Zero : simulink/Logic and Bit Operations/Compare To Zero  relop=<  OutDataTypeStr=boolean
  Compare To Zero1 : simulink/Logic and Bit Operations/Compare To Zero  relop=>=  OutDataTypeStr=boolean
  Delay6 : Delay  DelayLength=1
  Logical Operator : Logic  AllPortsSameDT=off  OutDataTypeStr=boolean
  Logical Operator17 : Logic  AllPortsSameDT=off  OutDataTypeStr=boolean
  Logical Operator18 : Logic  AllPortsSameDT=off  OutDataTypeStr=boolean
  zeroCrossingTrue : Outport
  wires:
  Logical Operator17/1 -> Logical Operator18/2
  Compare To Zero1/1 -> Logical Operator/2
  Logical Operator18/1 -> zeroCrossingTrue/1
  peakVal/1 -> Compare To Zero/1, Delay6/1
  Compare To Constant11/1 -> Logical Operator17/1
  Logical Operator/1 -> Logical Operator17/2
  Delay6/1 -> Compare To Zero1/1
  Compare To Zero/1 -> Logical Operator/1
  peakIndex/1 -> Compare To Constant11/1, Compare To Constant12/1
  Compare To Constant12/1 -> Logical Operator18/1

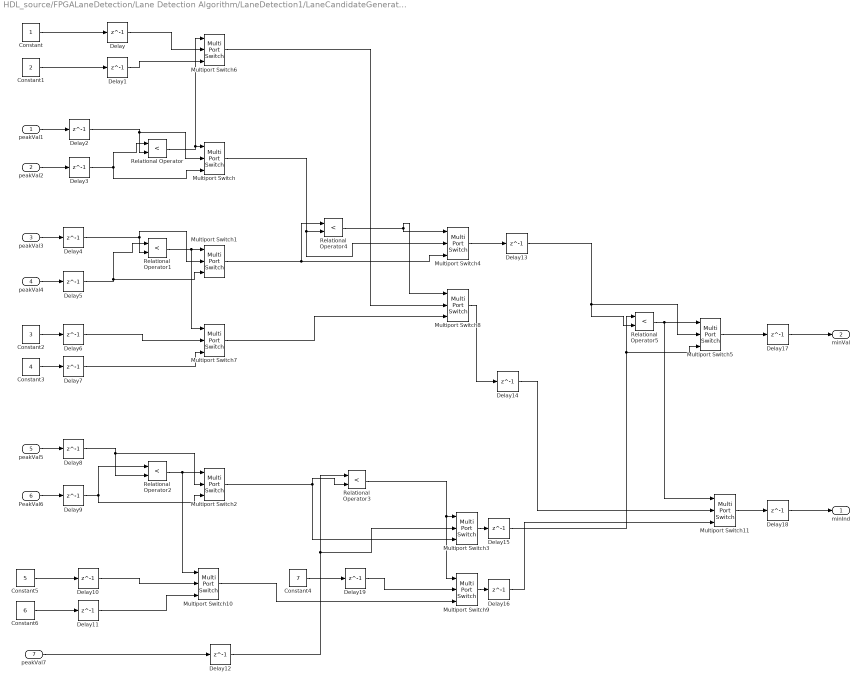
== system HDL_source/FPGALaneDetection/Lane Detection Algorithm/LaneDetection1/LaneCandidateGeneration/StoreDominantLanes/findMin ==
  peakVal1 : Inport
  peakVal2 : Inport  Port=2
  peakVal3 : Inport  Port=3
  peakVal4 : Inport  Port=4
  peakVal5 : Inport  Port=5
  PeakVal6 : Inport  Port=6
  peakVal7 : Inport  Port=7
  Constant : Constant  OutDataTypeStr=uint8  SampleTime=-1
  Constant1 : Constant  Value=2  OutDataTypeStr=uint8  SampleTime=-1
  Constant2 : Constant  Value=3  OutDataTypeStr=uint8  SampleTime=-1
  Constant3 : Constant  Value=4  OutDataTypeStr=uint8  SampleTime=-1
  Constant4 : Constant  Value=7  OutDataTypeStr=uint8  SampleTime=-1
  Constant5 : Constant  Value=5  OutDataTypeStr=uint8  SampleTime=-1
  Constant6 : Constant  Value=6  OutDataTypeStr=uint8  SampleTime=-1
  Delay{,1..19} (20 alike) : Delay  DelayLength=1
  Multiport Switch{,1..11} (12 alike) : MultiPortSwitch  DataPortOrder=Zero-based contiguous  Inputs=2  zeroidx=on
  Relational Operator{,1..5} (6 alike) : RelationalOperator  Operator=<  OutDataTypeStr=boolean  RndMeth=Nearest
  minInd : Outport
  minVal : Outport  Port=2
  wires:
  Delay19/1 -> Multiport Switch9/2
  Delay18/1 -> minInd/1
  Delay17/1 -> minVal/1
  Delay16/1 -> Multiport Switch11/3
  Delay15/1 -> Multiport Switch5/3, Relational Operator5/1
  Delay14/1 -> Multiport Switch11/2
  Delay13/1 -> Multiport Switch5/2, Relational Operator5/2
  Delay12/1 -> Multiport Switch3/2, Relational Operator3/1
  Delay11/1 -> Multiport Switch10/3
  Delay10/1 -> Multiport Switch10/2
  Delay9/1 -> Multiport Switch2/3, Relational Operator2/1
  Delay8/1 -> Relational Operator2/2, Multiport Switch2/2
  Delay7/1 -> Multiport Switch7/3
  Delay6/1 -> Multiport Switch7/2
  Delay5/1 -> Multiport Switch1/3, Relational Operator1/1
  Delay4/1 -> Relational Operator1/2, Multiport Switch1/2
  Delay3/1 -> Relational Operator/1, Multiport Switch/3
  Delay2/1 -> Relational Operator/2, Multiport Switch/2
  Delay1/1 -> Multiport Switch6/3
  Delay/1 -> Multiport Switch6/2
  Multiport Switch11/1 -> Delay18/1
  Multiport Switch9/1 -> Delay16/1
  Multiport Switch8/1 -> Delay14/1
  Multiport Switch10/1 -> Multiport Switch9/3
  Constant6/1 -> Delay11/1
  Constant5/1 -> Delay10/1
  Constant4/1 -> Delay19/1
  Multiport Switch7/1 -> Multiport Switch8/3
  Multiport Switch6/1 -> Multiport Switch8/2
  Constant2/1 -> Delay6/1
  Constant3/1 -> Delay7/1
  Constant1/1 -> Delay1/1
  Constant/1 -> Delay/1
  Multiport Switch5/1 -> Delay17/1
  Relational Operator5/1 -> Multiport Switch5/1, Multiport Switch11/1
  Multiport Switch3/1 -> Delay15/1
  Multiport Switch4/1 -> Delay13/1
  Multiport Switch1/1 -> Relational Operator4/1, Multiport Switch4/3
  Multiport Switch/1 -> Relational Operator4/2, Multiport Switch4/2
  Relational Operator4/1 -> Multiport Switch4/1, Multiport Switch8/1
  Relational Operator3/1 -> Multiport Switch3/1, Multiport Switch9/1
  Multiport Switch2/1 -> Multiport Switch3/3, Relational Operator3/2
  peakVal7/1 -> Delay12/1
  PeakVal6/1 -> Delay9/1
  peakVal5/1 -> Delay8/1
  Relational Operator2/1 -> Multiport Switch2/1, Multiport Switch10/1
  peakVal3/1 -> Delay4/1
  Relational Operator1/1 -> Multiport Switch1/1, Multiport Switch7/1
  Relational Operator/1 -> Multiport Switch/1, Multiport Switch6/1
  peakVal4/1 -> Delay5/1
  peakVal2/1 -> Delay3/1
  peakVal1/1 -> Delay2/1

== system HDL_source/FPGALaneDetection/Lane Detection Algorithm/LaneDetection1/LaneCandidateGeneration/StoreDominantLanes/peakValueMemory ==
  peakVal : Inport
  lane1En : Inport  Port=2
  lane3En : Inport  Port=3
  lane2En : Inport  Port=4
  lane4En : Inport  Port=5
  lane5En : Inport  Port=6
  lane6En : Inport  Port=7
  lane7En : Inport  Port=8
  laneRST : Inport  Port=9
  Delay{17..23} (7 alike) : Delay  DelayLength=1  ExternalReset=Level hold  ShowEnablePort=on
      settings: InputPortMap=u0,e6,r5
  peakREG1 : Outport
  peakREG2 : Outport  Port=2
  peakREG3 : Outport  Port=3
  peakREG4 : Outport  Port=4
  peakREG5 : Outport  Port=5
  peakREG6 : Outport  Port=6
  peakREG7 : Outport  Port=7
  wires:
  laneRST/1 -> Delay17/3, Delay18/3, Delay19/3, Delay20/3, Delay23/3, Delay22/3, Delay21/3
  Delay22/1 -> peakREG6/1
  lane5En/1 -> Delay21/2
  lane7En/1 -> Delay23/2
  Delay23/1 -> peakREG7/1
  Delay19/1 -> peakREG3/1
  Delay20/1 -> peakREG4/1
  lane2En/1 -> Delay18/2
  lane6En/1 -> Delay22/2
  lane1En/1 -> Delay17/2
  lane3En/1 -> Delay19/2
  lane4En/1 -> Delay20/2
  Delay21/1 -> peakREG5/1
  peakVal/1 -> Delay21/1, Delay22/1, Delay23/1, Delay20/1, Delay19/1, Delay18/1, Delay17/1
  Delay18/1 -> peakREG2/1
  Delay17/1 -> peakREG1/1

== system HDL_source/FPGALaneDetection/Lane Detection Algorithm/LaneDetection1/LaneCandidateGeneration/HistogramColumnCount/ColumnCountNeg/Subsystem ==
  Constant{,1..4} (5 alike) : Constant  Value=false  SampleTime=-1
  Pixel Control Bus Creator1 : visionhdlutilities/Pixel Control Bus Creator
      settings: SourceProductName=Vision HDL Toolbox  SourceProductBaseCode=VT
  Out1 : Outport
  wires:
  Constant3/1 -> Pixel Control Bus Creator1/4
  Constant4/1 -> Pixel Control Bus Creator1/5
  Pixel Control Bus Creator1/1 -> Out1/1
  Constant1/1 -> Pixel Control Bus Creator1/2
  Constant/1 -> Pixel Control Bus Creator1/1
  Constant2/1 -> Pixel Control Bus Creator1/3

== system HDL_source/FPGALaneDetection/Lane Detection Algorithm/LaneDetection1/LaneCandidateGeneration/HistogramColumnCount/ColumnCountNeg/Subsystem1 ==
  Constant{,1..4} (5 alike) : Constant  Value=false  SampleTime=-1
  Pixel Control Bus Creator1 : visionhdlutilities/Pixel Control Bus Creator
      settings: SourceProductName=Vision HDL Toolbox  SourceProductBaseCode=VT
  Out1 : Outport
  wires:
  Constant2/1 -> Pixel Control Bus Creator1/3
  Constant/1 -> Pixel Control Bus Creator1/1
  Constant1/1 -> Pixel Control Bus Creator1/2
  Pixel Control Bus Creator1/1 -> Out1/1
  Constant4/1 -> Pixel Control Bus Creator1/5
  Constant3/1 -> Pixel Control Bus Creator1/4

== system HDL_source/FPGALaneDetection/Lane Detection Algorithm/LaneDetection1/LaneCandidateGeneration/HistogramColumnCount/ColumnCountNeg/TiledROIExractor ==
  controlIn : Inport
  pixelIn : Inport  Port=2
  Compare To Constant1 : simulink/Logic and Bit Operations/Compare To Constant  relop===  const=0  OutDataTypeStr=boolean
  Compare To Constant2 : simulink/Logic and Bit Operations/Compare To Constant  relop===  const=27  OutDataTypeStr=boolean
  Constant : Constant  Value=0  OutDataTypeStr=fixdt(0,10,0)  SampleTime=-1
  Gain : Gain  Gain=1/2  OutDataTypeStr=fixdt(0,10,0)
  Logical Operator : Logic  AllPortsSameDT=off  OutDataTypeStr=boolean
  Logical Operator1 : Logic  Operator=OR  AllPortsSameDT=off  OutDataTypeStr=boolean
  Logical Operator2 : Logic  Operator=OR  AllPortsSameDT=off  OutDataTypeStr=boolean
  Logical Operator3 : Logic  AllPortsSameDT=off  OutDataTypeStr=boolean
  Logical Operator8 : Logic  AllPortsSameDT=off  OutDataTypeStr=boolean
  Pixel Control Bus Creator : visionhdlutilities/Pixel Control Bus Creator
      settings: SourceProductName=Vision HDL Toolbox  SourceProductBaseCode=VT
  Pixel Control Bus Selector : BusSelector  OutputSignals=hStart,hEnd,vStart,vEnd,valid
  Pixel Switch2 : MultiPortSwitch  DataPortOrder=Zero-based contiguous  Inputs=2  zeroidx=on
  RegionCount : hdlsllib/Sources/HDL Counter  CountType=Count limited  CountInit=0  CountStep=1  CountMax=40  CountFromType=Initial value  CountFrom=0  CountResetPort=on  CountLoadPort=off  CountEnbPort=on  CountDirPort=off  CountDataType=Unsigned  CountWordLen=6  CountFracLen=0  CountSampTime=1
      settings: SourceProductName=Simulink
  count pixels horizontally : hdlsllib/Sources/HDL Counter  CountType=Free running  CountInit=0  CountStep=1  CountMax=25  CountFromType=Initial value  CountFrom=0  CountResetPort=on  CountLoadPort=off  CountEnbPort=on  CountDirPort=off  CountDataType=Unsigned  CountWordLen=11  CountFracLen=0  CountSampTime=1
      settings: SourceProductName=Simulink
  regionStart : Outport
  pixelOut : Outport  Port=2
  controlOut : Outport  Port=3
  wires:
  Compare To Constant2/1 -> Logical Operator3/1
  Compare To Constant1/1 -> Logical Operator8/1
  controlIn/1 -> Pixel Control Bus Selector/1
  Pixel Control Bus Selector/5 -> count pixels horizontally/2, Logical Operator/2, Pixel Control Bus Creator/5  "<valid>"
  Pixel Control Bus Creator/1 -> controlOut/1
  Logical Operator2/1 -> RegionCount/1, regionStart/1, Pixel Control Bus Creator/4
  Pixel Control Bus Selector/3 -> Logical Operator1/2  "<vStart>"
  Logical Operator8/1 -> Logical Operator1/1
  Logical Operator1/1 -> Pixel Control Bus Creator/3
  count pixels horizontally/1 -> Gain/1
  Logical Operator3/1 -> Logical Operator2/2
  Pixel Switch2/1 -> pixelOut/1
  pixelIn/1 -> Logical Operator/1
  Logical Operator/1 -> Pixel Switch2/1
  Pixel Control Bus Selector/2 -> Pixel Control Bus Creator/2, Logical Operator3/2, count pixels horizontally/1  "<hEnd>"
  Pixel Control Bus Selector/1 -> Logical Operator8/2, Pixel Control Bus Creator/1, RegionCount/2  "<hStart>"
  Pixel Control Bus Selector/4 -> Logical Operator2/1  "<vEnd>"
  Constant/1 -> Pixel Switch2/2
  RegionCount/1 -> Compare To Constant1/1, Compare To Constant2/1
  Gain/1 -> Pixel Switch2/3

== system HDL_source/FPGALaneDetection/Lane Detection Algorithm/LaneDetection1/LaneCandidateGeneration/HistogramColumnCount/ColumnCountPos/Subsystem ==
  Constant{,1..4} (5 alike) : Constant  Value=false  SampleTime=-1
  Pixel Control Bus Creator1 : visionhdlutilities/Pixel Control Bus Creator
      settings: SourceProductName=Vision HDL Toolbox  SourceProductBaseCode=VT
  Out1 : Outport
  wires:
  Constant2/1 -> Pixel Control Bus Creator1/3
  Constant/1 -> Pixel Control Bus Creator1/1
  Constant1/1 -> Pixel Control Bus Creator1/2
  Pixel Control Bus Creator1/1 -> Out1/1
  Constant4/1 -> Pixel Control Bus Creator1/5
  Constant3/1 -> Pixel Control Bus Creator1/4

== system HDL_source/FPGALaneDetection/Lane Detection Algorithm/LaneDetection1/LaneCandidateGeneration/HistogramColumnCount/ColumnCountPos/Subsystem1 ==
  Constant{,1..4} (5 alike) : Constant  Value=false  SampleTime=-1
  Pixel Control Bus Creator1 : visionhdlutilities/Pixel Control Bus Creator
      settings: SourceProductName=Vision HDL Toolbox  SourceProductBaseCode=VT
  Out1 : Outport
  wires:
  Constant3/1 -> Pixel Control Bus Creator1/4
  Constant4/1 -> Pixel Control Bus Creator1/5
  Pixel Control Bus Creator1/1 -> Out1/1
  Constant1/1 -> Pixel Control Bus Creator1/2
  Constant/1 -> Pixel Control Bus Creator1/1
  Constant2/1 -> Pixel Control Bus Creator1/3

== system HDL_source/FPGALaneDetection/Lane Detection Algorithm/LaneDetection1/LaneCandidateGeneration/HistogramColumnCount/ColumnCountPos/TiledROIExractor ==
  controlIn : Inport
  pixelIn : Inport  Port=2
  Compare To Constant1 : simulink/Logic and Bit Operations/Compare To Constant  relop===  const=0  OutDataTypeStr=boolean
  Compare To Constant2 : simulink/Logic and Bit Operations/Compare To Constant  relop===  const=27  OutDataTypeStr=boolean
  Constant : Constant  Value=0  OutDataTypeStr=fixdt(0,10,0)  SampleTime=-1
  Gain : Gain  Gain=1/2  OutDataTypeStr=fixdt(0,10,0)
  Logical Operator : Logic  AllPortsSameDT=off  OutDataTypeStr=boolean
  Logical Operator1 : Logic  Operator=OR  AllPortsSameDT=off  OutDataTypeStr=boolean
  Logical Operator2 : Logic  Operator=OR  AllPortsSameDT=off  OutDataTypeStr=boolean
  Logical Operator3 : Logic  AllPortsSameDT=off  OutDataTypeStr=boolean
  Logical Operator8 : Logic  AllPortsSameDT=off  OutDataTypeStr=boolean
  Pixel Control Bus Creator : visionhdlutilities/Pixel Control Bus Creator
      settings: SourceProductName=Vision HDL Toolbox  SourceProductBaseCode=VT
  Pixel Control Bus Selector : BusSelector  OutputSignals=hStart,hEnd,vStart,vEnd,valid
  Pixel Switch2 : MultiPortSwitch  DataPortOrder=Zero-based contiguous  Inputs=2  zeroidx=on
  RegionCount : hdlsllib/Sources/HDL Counter  CountType=Count limited  CountInit=0  CountStep=1  CountMax=40  CountFromType=Initial value  CountFrom=0  CountResetPort=on  CountLoadPort=off  CountEnbPort=on  CountDirPort=off  CountDataType=Unsigned  CountWordLen=6  CountFracLen=0  CountSampTime=1
      settings: SourceProductName=Simulink
  count pixels horizontally : hdlsllib/Sources/HDL Counter  CountType=Free running  CountInit=0  CountStep=1  CountMax=25  CountFromType=Initial value  CountFrom=0  CountResetPort=on  CountLoadPort=off  CountEnbPort=on  CountDirPort=off  CountDataType=Unsigned  CountWordLen=11  CountFracLen=0  CountSampTime=1
      settings: SourceProductName=Simulink
  regionStart : Outport
  pixelOut : Outport  Port=2
  controlOut : Outport  Port=3
  wires:
  Compare To Constant2/1 -> Logical Operator3/1
  Compare To Constant1/1 -> Logical Operator8/1
  controlIn/1 -> Pixel Control Bus Selector/1
  Pixel Control Bus Selector/5 -> count pixels horizontally/2, Logical Operator/2, Pixel Control Bus Creator/5  "<valid>"
  Pixel Control Bus Creator/1 -> controlOut/1
  Logical Operator2/1 -> RegionCount/1, regionStart/1, Pixel Control Bus Creator/4
  Pixel Control Bus Selector/3 -> Logical Operator1/2  "<vStart>"
  Logical Operator8/1 -> Logical Operator1/1
  Logical Operator1/1 -> Pixel Control Bus Creator/3
  count pixels horizontally/1 -> Gain/1
  Logical Operator3/1 -> Logical Operator2/2
  Pixel Switch2/1 -> pixelOut/1
  pixelIn/1 -> Logical Operator/1
  Logical Operator/1 -> Pixel Switch2/1
  Pixel Control Bus Selector/2 -> Pixel Control Bus Creator/2, Logical Operator3/2, count pixels horizontally/1  "<hEnd>"
  Pixel Control Bus Selector/1 -> Logical Operator8/2, Pixel Control Bus Creator/1, RegionCount/2  "<hStart>"
  Pixel Control Bus Selector/4 -> Logical Operator2/1  "<vEnd>"
  Constant/1 -> Pixel Switch2/2
  RegionCount/1 -> Compare To Constant1/1, Compare To Constant2/1
  Gain/1 -> Pixel Switch2/3

== matlab function HDL_source/SWLaneFitandOverlay/Driver ==
  data: dataReady input; swStart output; process output; swDone input
function [swStart,process] = fcn(dataReady,swDone)

persistent FSMState;

% define states
S0 = uint8(0);
S1 = uint8(1);
S2 = uint8(2);

if isempty(FSMState) 
   FSMState = S0; 
end

switch FSMState
    case S0 %software polling 
        if dataReady
            FSMState = S1;
            swStart =  true;
            process = true;         
        else
            FSMState = S0;
            swStart =  true;
            process = false;        
        end
                       
    case S1 % software processing
        if swDone
            FSMState = S2;
            swStart =  false;
            process = false;                    
        else
            FSMState = S1;
            swStart =  true;
            process = true;
        end
      
    case S2 % synchronize with hardware
        if ~dataReady
            FSMState = S0;
            swStart =  true;
            process = false;                    
        else
            FSMState = S2;
            swStart =  false;
            process = false;                    
        end
      
    otherwise
        swStart =  false;
        process = false;
        FSMState = S0;
end

end
